simulink model "leader_qball2_mytest"  (R2014a)
settings: Solver=ode1  StartTime=0.0  StopTime=inf  FixedStep=0.002  RelTol=1e-3
InitFcn:
  | QBall_2_Setup
values from neighbouring files (symbols this model uses):
  g = 9.81    [QBall_2_System_Parameters.m]
  joystick_range_max = 0.8    [QBall_2_Setup.m]
  joystick_range_min = 0.5    [QBall_2_Setup.m]
  KdHEIGHT_DOWN = 0.15    [QBall_2_Controller_Design.m]
  KdHEIGHT_UP = 0.15    [QBall_2_Controller_Design.m]
  KdOUTER_PITCH_DOWN = 0.4    [QBall_2_Controller_Design.m]
  KdOUTER_PITCH_UP = 0.6    [QBall_2_Controller_Design.m]
  KdOUTER_ROLL_DOWN = 0.4    [QBall_2_Controller_Design.m]
  KdOUTER_ROLL_UP = 0.4    [QBall_2_Controller_Design.m]
  KdPITCH_DOWN = 0.1    [QBall_2_Controller_Design.m]
  KdPITCH_UP = 0.1    [QBall_2_Controller_Design.m]
  KdROLL_DOWN = 0.1    [QBall_2_Controller_Design.m]
  KdROLL_UP = 0.1    [QBall_2_Controller_Design.m]
  KdYAW_DOWN = 0.32    [QBall_2_Controller_Design.m]
  KdYAW_UP = 0.32    [QBall_2_Controller_Design.m]
  KiHEIGHT_DOWN = 0.35    [QBall_2_Controller_Design.m]
  KiHEIGHT_UP = 0.35    [QBall_2_Controller_Design.m]
  KiOUTER_PITCH_DOWN = 0.08    [QBall_2_Controller_Design.m]
  KiOUTER_PITCH_UP = 0.08    [QBall_2_Controller_Design.m]
  KiOUTER_ROLL_DOWN = 0.08    [QBall_2_Controller_Design.m]
  KiOUTER_ROLL_UP = 0.08    [QBall_2_Controller_Design.m]
  KiPITCH_DOWN = 0.08    [QBall_2_Controller_Design.m]
  KiPITCH_UP = 0.08    [QBall_2_Controller_Design.m]
  KiROLL_DOWN = 0.08    [QBall_2_Controller_Design.m]
  KiROLL_UP = 0.08    [QBall_2_Controller_Design.m]
  KiYAW_DOWN = 0.0    (= 0)    [QBall_2_Controller_Design.m]
  KiYAW_UP = 0.0    (= 0)    [QBall_2_Controller_Design.m]
  KpHEIGHT_DOWN = 0.5    [QBall_2_Controller_Design.m]
  KpHEIGHT_UP = 0.5    [QBall_2_Controller_Design.m]
  KpOUTER_PITCH_DOWN = 0.3    [QBall_2_Controller_Design.m]
  KpOUTER_PITCH_UP = 0.3    [QBall_2_Controller_Design.m]
  KpOUTER_ROLL_DOWN = 0.3    [QBall_2_Controller_Design.m]
  KpOUTER_ROLL_UP = 0.3    [QBall_2_Controller_Design.m]
  KpPITCH_DOWN = 0.5    [QBall_2_Controller_Design.m]
  KpPITCH_UP = 0.5    [QBall_2_Controller_Design.m]
  KpROLL_DOWN = 0.5    [QBall_2_Controller_Design.m]
  KpROLL_UP = 0.5    [QBall_2_Controller_Design.m]
  KpYAW_DOWN = 0.45    [QBall_2_Controller_Design.m]
  KpYAW_UP = 0.45    [QBall_2_Controller_Design.m]
  LIMIT_CMD_PITCH = 5*pi/180    (= 0.0872664625997)    [QBall_2_Controller_Design.m]
  LIMIT_CMD_ROLL = 5*pi/180    (= 0.0872664625997)    [QBall_2_Controller_Design.m]
  LIMIT_MAX_HEIGHT = 2    [QBall_2_Controller_Design.m]
  LIMIT_MAX_X = 1    [QBall_2_Controller_Design.m]
  LIMIT_MAX_Z = 1    [QBall_2_Controller_Design.m]
  LIMIT_MIN_HEIGHT = 0.3    [QBall_2_Controller_Design.m]
  LIMIT_MIN_X = -1    [QBall_2_Controller_Design.m]
  LIMIT_MIN_Z = -1    [QBall_2_Controller_Design.m]
  LIMIT_RATE_HEIGHT = 0.05    [QBall_2_Controller_Design.m]
  LIMIT_RATE_X = 0.15    [QBall_2_Controller_Design.m]
  LIMIT_RATE_YAW = 15*pi/180    (= 0.261799387799)    [QBall_2_Controller_Design.m]
  LIMIT_RATE_Z = 0.15    [QBall_2_Controller_Design.m]
  LIMIT_uCMD_PITCH = 0.5    [QBall_2_Controller_Design.m]
  LIMIT_uCMD_ROLL = 0.5    [QBall_2_Controller_Design.m]
  LIMIT_uCMD_YAW = 0.5    [QBall_2_Controller_Design.m]
  OFFSET_HEIGHT = 0.3    [QBall_2_System_Parameters.m]
  OMEGA_FILTER = 60    [QBall_2_System_Parameters.m]
  TRIM_THROTTLE = M*g/(4*K)    [QBall_2_Controller_Design.m]
  TRIM_U_PITCH = 0.009    [QBall_2_Controller_Design.m]
  TRIM_U_ROLL = -0.0065    [QBall_2_Controller_Design.m]
undefined symbols (not defined in the file or in its folder): DiscIntNeverNeededParam, qc_get_step_size
libraries: simulink x27, quarc_library x27
(part 3 of 3)

== matlab function leader_qball2_mytest/DAQ/Initialize sensors/Sensor Fusion//Filtering/Kalman Filter - Roll ==
  data: angle output; acc_angle input; gyro_rate input; dt input; BatteryOnTop input
function angle   = fcn(acc_angle,gyro_rate,dt,BatteryOnTop)
%#eml

    if(BatteryOnTop == 1)
        Q_angle  = 0.001; %0.01; %0.001
    else
        Q_angle = 0.01;
    end;
    Q_gyro   = 0.01; %0.01;  %0.003
    R_angle  =  0.03;  %0.03

    
    persistent P_00;
    persistent P_01;
    persistent P_10;
    persistent P_11;
    persistent x_angle;
    persistent x_bias;
        
    if isempty(P_00)
        P_00 = 0;
    end
    
    if isempty(P_01)
        P_01 = 0;
    end
    if isempty(P_10)
        P_10 = 0;
    end
    if isempty(P_11)
        P_11 = 0;
    end
     if isempty(x_bias)
        x_bias = 0;
     end
     if isempty(x_angle)
        x_angle = 0;
     end
    
    
    % Calculate the new output
    x_angle = x_angle + dt * (gyro_rate - x_bias);
    P_00 = P_00 -  dt * (P_10 + P_01) + Q_angle * dt;
    P_01 = P_01  - dt * P_11;
    P_10 = P_10  - dt * P_11;
    P_11 = P_11  + Q_gyro * dt;

    % Assuming H = [0.97 (effect of gyro) 0.03 (effect of acc)]
    e = (0.97*x_angle + 0.03*acc_angle) - x_angle;
    S = P_00 + R_angle;
    K_0 = P_00 / S;
    K_1 = P_10 / S;

    % Correction
    x_angle = x_angle+  K_0 * e;
    x_bias  = x_bias+  K_1 * e;
    P_00 = P_00 - K_0 * P_00;
    P_01 = P_01 - K_0 * P_01;
    P_10 = P_10 - K_1 * P_00;
    P_11 = P_11 - K_1 * P_01;

    angle = x_angle;

== matlab function leader_qball2_mytest/Roll Controller/Subsystem/OT pos control/adjust_for_heading/adjust_roll_command ==
  data: roll_cmd input; adj_roll_cmd output; pitch_cmd input; heading input
function adj_roll_cmd = fcn(roll_cmd, pitch_cmd, heading)
%#eml

% Given the roll and pitch commands computed for the global frame, this function
% rotates the roll command into the local frame, allowing the control
% command to work even for non-zero yaw.

adj_roll_cmd = roll_cmd*cos(heading) + pitch_cmd*sin(heading);
%adj_roll_cmd = roll_cmd*cos(heading) - pitch_cmd*sin(heading);

== matlab function leader_qball2_mytest/Pitch Controller/Subsystem/OT pos control/adjust_for_heading/adjust_pitch_command ==
  data: pitch_cmd input; roll_cmd input; adj_pitch_cmd output; heading input
function adj_pitch_cmd = fcn(pitch_cmd, roll_cmd, heading)
%#eml

% Given the roll and pitch commands computed for the global frame, this function
% rotates the pitch command into the local frame, allowing the control
% command to work even for non-zero yaw.

adj_pitch_cmd = -roll_cmd*sin(heading) + pitch_cmd*cos(heading);
%adj_pitch_cmd = roll_cmd*sin(heading) + pitch_cmd*cos(heading);

== matlab function leader_qball2_mytest/DAQ/Initialize sensors/Sensor Fusion//Filtering/Kalman Filter - Yaw ==
  data: angle output; acc_angle input; gyro_rate input; dt input
function angle   = fcn(acc_angle,gyro_rate,dt)
%#eml

     Q_angle  = 0.01; %0.01; %0.001
     Q_gyro   = 0.01; %0.01;  %0.003
     R_angle  =  0.03;  %0.03

    
    persistent P_00;
    persistent P_01;
    persistent P_10;
    persistent P_11;
    persistent x_angle;
    persistent x_bias;
        
    if isempty(P_00)
        P_00 = 0;
    end
    
    if isempty(P_01)
        P_01 = 0;
    end
    if isempty(P_10)
        P_10 = 0;
    end
    if isempty(P_11)
        P_11 = 0;
    end
     if isempty(x_bias)
        x_bias = 0;
     end
     if isempty(x_angle)
        x_angle = 0;
     end
    
    
    % Calculate the new output
    x_angle = x_angle + dt * (gyro_rate - x_bias);
    P_00 = P_00 -  dt * (P_10 + P_01) + Q_angle * dt;
    P_01 = P_01  - dt * P_11;
    P_10 = P_10  - dt * P_11;
    P_11 = P_11  + Q_gyro * dt;

    % Assuming H = [0.98 (effect of gyro) 0.02 (effect of acc)]
    e = (0.5*x_angle + 0.5*acc_angle) - x_angle;
    S = P_00 + R_angle;
    K_0 = P_00 / S;
    K_1 = P_10 / S;

    % Correction
    x_angle = x_angle+  K_0 * e;
    x_bias  = x_bias+  K_1 * e;
    P_00 = P_00 - K_0 * P_00;
    P_01 = P_01 - K_0 * P_01;
    P_10 = P_10 - K_1 * P_00;
    P_11 = P_11 - K_1 * P_01;

    angle = x_angle;

== matlab function leader_qball2_mytest/DAQ/Initialize sensors/Sensor Fusion//Filtering/Calculate Roll and Pitch (From Acceleration Data)/calc_roll_pitch ==
  data: roll_acc output; pitch_acc output; acc_body input
function [roll_acc, pitch_acc]   = fcn(acc_body)
%#eml
n = norm(acc_body,2);
if n>eps
    acc_body = -acc_body/n; 
else
    acc_body = [0 0 1]';
end

roll_acc = atan2(acc_body(2),acc_body(3));
pitch_acc = atan2( -acc_body(1), acc_body(2)*sin(roll_acc)+acc_body(3)*cos(roll_acc));

== matlab function leader_qball2_mytest/DAQ/Initialize sensors/Sensor Fusion//Filtering/Kalman Filter - Height ==
  data: height output; optitrack input; sonar_d input; dt input
function height   = fcn(optitrack,sonar_d,dt)
%#eml

     Q_sonar  = 0.1; %0.01; %0.001
     Q_optitrack   = 0.01; %0.01;  %0.003
     R_height =  0.03;  %0.03

    
    persistent P_00;
    persistent P_01;
    persistent P_10;
    persistent P_11;
    persistent x_height;
    persistent x_bias;
        
    if isempty(P_00)
        P_00 = 0;
    end
    
    if isempty(P_01)
        P_01 = 0;
    end
    if isempty(P_10)
        P_10 = 0;
    end
    if isempty(P_11)
        P_11 = 0;
    end
     if isempty(x_bias)
        x_bias = 0;
     end
     if isempty(x_height)
        x_height = 0;
     end
    
    
    % Calculate the new output
    x_height = x_height + dt * (sonar_d - x_bias);
    P_00 = P_00 -  dt * (P_10 + P_01) + Q_sonar * dt;
    P_01 = P_01  - dt * P_11;
    P_10 = P_10  - dt * P_11;
    P_11 = P_11  + Q_optitrack * dt;

    % Assuming H = [0.95 (effect of optitrack) 0.05 (effect of sonar)]
    e = (0.05*x_height + 0.95*optitrack) - x_height;
    S = P_00 + R_height;
    K_0 = P_00 / S;
    K_1 = P_10 / S;

    % Correction
    x_height = x_height+  K_0 * e;
    x_bias  = x_bias+  K_1 * e;
    P_00 = P_00 - K_0 * P_00;
    P_01 = P_01 - K_0 * P_01;
    P_10 = P_10 - K_1 * P_00;
    P_11 = P_11 - K_1 * P_01;

    height = x_height;

== matlab function leader_qball2_mytest/DAQ/Initialize sensors/Nonlinear Limit (Reject Spikes)/Embedded MATLAB Function ==
  data: u input; y output; x input; threshold input
function y = fcn(u,x,threshold)
% This block supports the Embedded MATLAB subset.
% See the help menu for details. 

if (abs(u-x)<threshold)
    y = u;
else
    y = x;
end

== matlab function leader_qball2_mytest/DAQ/Initialize sensors/Calibrate Accelerometer Data/correct accel mounting ==
  data: u input; n output; nhat output; Phi output; Theta output; check output; R output; acc input; acc_body output
function [n,nhat,Phi,Theta,check, R, acc_body]   = fcn(u,acc)
%#eml

n = norm(u,2);

if n>eps
    nhat = -u/n;
else
    nhat = [0 0 1]';
end
    
Phi = atan2(nhat(2),nhat(3));
Theta = atan2 (-nhat(1),(nhat(2)*sin(Phi)+nhat(3)*cos(Phi)));

sPhi = sin(Phi);
cPhi = cos(Phi);

sTheta = sin(Theta);
cTheta = cos(Theta);



check = -sin(Theta)*nhat(1)+sin(Phi)*cos(Theta)*nhat(2)+cos(Phi)*cos(Theta)*nhat(3);


R = [cTheta, sPhi*sTheta, cPhi*sTheta
    0,  cPhi,  -sPhi
    -sTheta,  sPhi*cTheta,  cPhi*cTheta];

acc_body = R*acc;

== matlab function leader_qball2_mytest/DAQ/Initialize sensors/Sensor Fusion//Filtering/Calculate Roll and Pitch (From Acceleration Data)/calc_roll_pitch_asin ==
  data: roll_acc output; pitch_acc output; acc_body input
function [roll_acc, pitch_acc]   = fcn(acc_body)
%#eml

roll_acc = asin(-acc_body(2)/9.8);

pitch_acc = asin(acc_body(1)/9.8);
